simulink model "Complex_Model"  (R2018b)
settings: Solver=ode45  StartTime=0.0  StopTime=10.0  RelTol=1e-3  EnableMultiTasking=on
PreLoadFcn:
  | load Buses
libraries: CustomLibrary x4, CustomLib x4
settings Model: Creator=Rose  LastModifiedBy=Rose
settings DataIOCC: LimitDataPoints=on  SaveFormat=Array  SignalLoggingSaveFormat=ModelDataLogs
settings OptimizationCC: ExpressionDepthLimit=2147483647  LifeSpan=inf
settings DebuggingCC: UnderspecifiedInitializationDetection=Classic  MergeDetectMultiDrivingBlocksExec=none  SolverPrmCheckMsg=warning  FcnCallInpInsideContextMsg=warning  AllowSymbolicDim=off  StateNameClashWarn=warning  LibraryContextMissingDiagnostic=none  SFUnexpectedBacktrackingDiag=warning  SFNoUnconditionalDefaultTransitionDiag=warning  SFExecutionAtInitializationDiag=none
settings HardwareCC: ProdBitPerPointer=32  ProdBitPerSizeT=32  ProdBitPerPtrDiffT=32  ProdLargestAtomicFloat=None  ProdIntDivRoundTo=Undefined  ProdEndianess=Unspecified  ProdWordSize=32  ProdHWDeviceType=32-bit Generic
settings ModelReferenceCC: PropagateSignalLabelsOutOfModel=off
settings SFSimCC: SimUseLocalCustomCode=off
settings RTWCC: RTWUseLocalCustomCode=off
settings CodeAppCC: StateflowObjectComments=on
settings GRTTargetCC: TargetLangStandard=C89/C90 (ANSI)  GeneratePreprocessorConditionals=Disable all  CombineOutputUpdateFcns=off  GRTInterface=on
settings ConfigComp: CovMetricSettings=dw  CovHtmlReporting=on  CovSaveCumulativeToWorkspaceVar=on  CovSaveSingleToWorkspaceVar=on  CovExternalEMLEnable=off

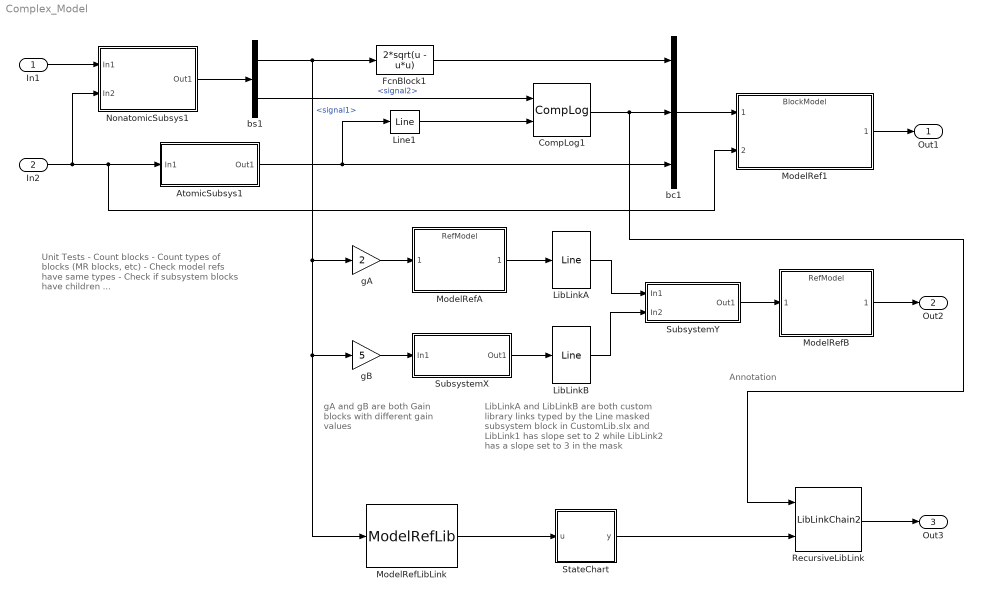
== system Complex_Model ==
  note: Unit Tests
      | - Count blocks
      | - Count types of blocks (MR blocks, etc)
      | - Check model refs have same types
      | - Check if subsystem blocks have children
      | ...
  note: Annotation
  note: LibLinkA and LibLinkB are both custom library links typed by the Line masked subsystem block in CustomLib.slx and LibLink1 has slope set to 2 while LibLink2 has a slope set to 3 in the mask
  note: gA and gB are both Gain blocks with different gain values
  In1 : Inport  OutDataTypeStr=Bus: Bus_1  SampleTime=[0,1]
  In2 : Inport  Port=2  OutDataTypeStr=int32  SampleTime=[0,1]
  AtomicSubsys1 : Subsystem  TreatAsAtomicUnit=on
  CompLog1 : CustomLibrary/CompLog  SystemSampleTime=-1
  FcnBlock1 : Fcn  Expr=2*sqrt(u - u*u)
  LibLinkA : CustomLib/MaskedSubsystems/Line  m=2  b=-1
  LibLinkB : CustomLib/MaskedSubsystems/Line  m=3  b=-1
  Line1 : CustomLibrary/Line  m=2  b=-1
  ModelRef1 : ModelReference  ModelNameDialog=BlockModel  SimulationMode=Normal  ModelReferenceVersion=1.41
  ModelRefA : ModelReference  ModelNameDialog=RefModel  SimulationMode=Normal  ModelReferenceVersion=1.38
  ModelRefB : ModelReference  ModelNameDialog=RefModel  SimulationMode=Normal  ModelReferenceVersion=1.38
  ModelRefLibLink : CustomLib/MaskedMRBlocks/ModelRefLib  ModelNameDialog=RefModel  SimulationMode=Normal  ShowModelInitializePort=off  ShowModelResetPorts=off  ShowModelTerminatePort=off  ShowModelPeriodicEventPorts=off  CodeInterface=Model reference  ModelReferenceVersion=1.38
  NonatomicSubsys1 : Subsystem
  RecursiveLibLink : CustomLib/MaskedCustomLibLink/LibLinkChain2  SystemSampleTime=-1
  StateChart : Stateflow chart  TreatAsAtomicUnit=on
  SubsystemX : Subsystem
  SubsystemY : Subsystem
  bc1 : BusCreator  Inputs=3  OutDataTypeStr=Bus: Bus_2
  bs1 : BusSelector  OutputSignals=signal1,signal2
  gA : Gain  Gain=2
  gB : Gain  Gain=5
  Out1 : Outport  OutDataTypeStr=Bus: Bus_1
  Out2 : Outport  Port=2  OutDataTypeStr=double
  Out3 : Outport  Port=3  OutDataTypeStr=boolean
  wires:
  In1/1 -> NonatomicSubsys1/1(In1)
  In2/1 -> NonatomicSubsys1/2(In2), AtomicSubsys1/1(In1), ModelRef1/2
  ModelRef1/1 -> Out1/1
  NonatomicSubsys1/1(Out1) -> bs1/1
  bc1/1 -> ModelRef1/1
  AtomicSubsys1/1(Out1) -> Line1/1, bc1/3
  bs1/1 -> ModelRefLibLink/1, gB/1, gA/1, FcnBlock1/1  "<signal1>"
  bs1/2 -> CompLog1/1  "<signal2>"
  FcnBlock1/1 -> bc1/1
  CompLog1/1 -> RecursiveLibLink/1, bc1/2
  Line1/1 -> CompLog1/2
  SubsystemY/1(Out1) -> ModelRefB/1
  SubsystemX/1(Out1) -> LibLinkB/1
  gB/1 -> SubsystemX/1(In1)
  LibLinkB/1 -> SubsystemY/2(In2)
  LibLinkA/1 -> SubsystemY/1(In1)
  gA/1 -> ModelRefA/1
  ModelRefA/1 -> LibLinkA/1
  ModelRefB/1 -> Out2/1
  RecursiveLibLink/1 -> Out3/1
  ModelRefLibLink/1 -> StateChart/1(u)
  StateChart/1(y) -> RecursiveLibLink/2

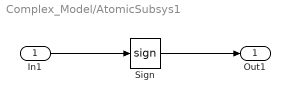
== system Complex_Model/AtomicSubsys1 ==
  In1 : Inport  OutDataTypeStr=int32
  Sign : Signum
  Out1 : Outport  OutDataTypeStr=int32
  wires:
  In1/1 -> Sign/1
  Sign/1 -> Out1/1

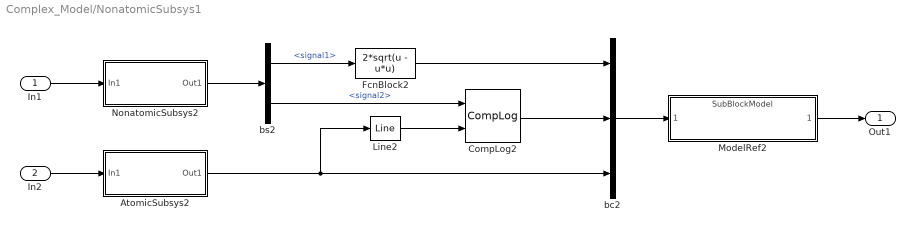
== system Complex_Model/NonatomicSubsys1 ==
  In1 : Inport  OutDataTypeStr=Bus: Bus_1
  In2 : Inport  Port=2  OutDataTypeStr=int32  SampleTime=[0,1]
  AtomicSubsys2 : Subsystem  TreatAsAtomicUnit=on
  CompLog2 : CustomLibrary/CompLog  SystemSampleTime=-1
  FcnBlock2 : Fcn  Expr=2*sqrt(u - u*u)
  Line2 : CustomLibrary/Line  m=2  b=-1
  ModelRef2 : ModelReference  ModelNameDialog=SubBlockModel  SimulationMode=Normal  ModelReferenceVersion=1.41
  NonatomicSubsys2 : Subsystem
  bc2 : BusCreator  Inputs=3  OutDataTypeStr=Bus: Bus_2
  bs2 : BusSelector  OutputSignals=signal1,signal2
  Out1 : Outport  OutDataTypeStr=Bus: Bus_1
  wires:
  In1/1 -> NonatomicSubsys2/1(In1)
  In2/1 -> AtomicSubsys2/1(In1)
  ModelRef2/1 -> Out1/1
  NonatomicSubsys2/1(Out1) -> bs2/1
  bc2/1 -> ModelRef2/1
  AtomicSubsys2/1(Out1) -> Line2/1, bc2/3
  bs2/1 -> FcnBlock2/1  "<signal1>"
  bs2/2 -> CompLog2/1  "<signal2>"
  FcnBlock2/1 -> bc2/1
  CompLog2/1 -> bc2/2
  Line2/1 -> CompLog2/2

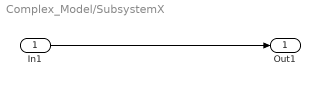
== system Complex_Model/SubsystemX ==
  In1 : Inport  OutDataTypeStr=double
  Out1 : Outport  OutDataTypeStr=double
  wires:
  In1/1 -> Out1/1

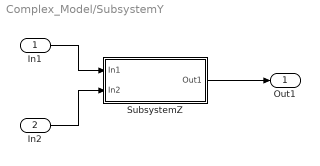
== system Complex_Model/SubsystemY ==
  In1 : Inport  OutDataTypeStr=double
  In2 : Inport  Port=2  OutDataTypeStr=double
  SubsystemZ : Subsystem
  Out1 : Outport  OutDataTypeStr=double
  wires:
  In2/1 -> SubsystemZ/2(In2)
  SubsystemZ/1(Out1) -> Out1/1
  In1/1 -> SubsystemZ/1(In1)

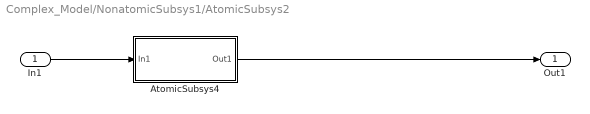
== system Complex_Model/NonatomicSubsys1/AtomicSubsys2 ==
  In1 : Inport  OutDataTypeStr=int32
  AtomicSubsys4 : Subsystem  TreatAsAtomicUnit=on
  Out1 : Outport  OutDataTypeStr=int32
  wires:
  In1/1 -> AtomicSubsys4/1(In1)
  AtomicSubsys4/1(Out1) -> Out1/1

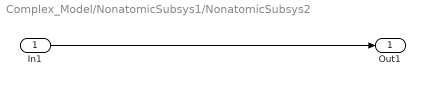
== system Complex_Model/NonatomicSubsys1/NonatomicSubsys2 ==
  In1 : Inport  OutDataTypeStr=Bus: Bus_1
  Out1 : Outport  OutDataTypeStr=Bus: Bus_1
  wires:
  In1/1 -> Out1/1

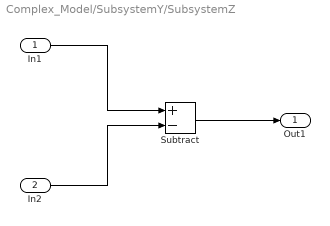
== system Complex_Model/SubsystemY/SubsystemZ ==
  In1 : Inport  OutDataTypeStr=double
  In2 : Inport  Port=2  OutDataTypeStr=double
  Subtract : Sum  Inputs=+-
  Out1 : Outport  OutDataTypeStr=double
  wires:
  Subtract/1 -> Out1/1
  In1/1 -> Subtract/1
  In2/1 -> Subtract/2

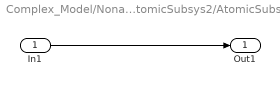
== system Complex_Model/NonatomicSubsys1/AtomicSubsys2/AtomicSubsys4 ==
  In1 : Inport  OutDataTypeStr=int32
  Out1 : Outport  OutDataTypeStr=int32
  wires:
  In1/1 -> Out1/1

== stateflow chart Complex_Model/StateChart ==
  state ON
    entry: y = 1;
  state OFF
    entry: y = -1;
  (default) -> ON
  ON -> OFF : [u<0]
  OFF -> ON : [u>0]
  data: u input; y output
